simulink model "threeDOF"  (R2019b)
settings: Solver=ode3  StartTime=0.0  StopTime=inf  FixedStep=0.05  RelTol=1e-3  EnableMultiTasking=on
model workspace (MAT data in the model file):
  m = Simulink.Parameter
  m.Value = 2000
  m.DataType = 'auto'
  m.Dimensions = [1 1]
undefined symbols (not defined in the file): Angular, FrameId, FrameId_SL_Info, Linear, Seq, Stamp, X, Y, Z
libraries: robotlib x30, eeGeneralControl x1, vehdynlibsteering x1, autolibshared x1, sharedtransform x1
settings Model: ExplicitPartitioning=on  Creator=ivory  LastModifiedBy=ivory
settings DataIOCC: ReturnWorkspaceOutputs=off
settings OptimizationCC: StrengthReduction=on  PassReuseOutputArgsAs=Individual arguments  MaxStackSize=64  OptimizeBlockOrder=speed  OptimizationPriority=Speed  OptimizationCustomize=off  MultiThreadedLoops=on  EfficientTunableParamExpr=on
settings DebuggingCC: ParameterTunabilityLossMsg=error  ArithmeticOperatorsInVariantConditions=warning
settings HardwareCC: ProdBitPerPointer=32  ProdBitPerSizeT=32  ProdBitPerPtrDiffT=32  ProdLargestAtomicFloat=None  ProdIntDivRoundTo=Undefined  ProdEndianess=Unspecified  ProdWordSize=32  ProdHWDeviceType=Generic->Unspecified (assume 32-bit Generic)
settings SFSimCC: MATLABDynamicMemAlloc=off  CustomCodeUndefinedFunction=UseInterfaceOnly
settings RTWCC: SystemTargetFile=ert.tlc  HardwareBoard=Robot Operating System (ROS)  TLCOptions="-aInlineSetEventsForThisBaseRateFcn=TLC_FALSE -aSuppressMultiTaskScheduler=TLC_FALSE  -aRateBasedStepFcn=0"  TemplateMakefile=ert_default_tmf  GenerateReport=on  Toolchain=Catkin  IncludeHyperlinkInReport=on  LaunchReport=on  TargetLang=C++  GenerateTraceInfo=on  GenerateTraceReport=on  GenerateTraceReportSl=on  GenerateTraceReportSf=on  GenerateTraceReportEml=on
settings CodeAppCC: ForceParamTrailComments=on  IgnoreCustomStorageClasses=off  OperatorAnnotations=on  SimulinkDataObjDesc=on  SFDataObjDesc=on  InsertBlockDesc=on
settings ERTTargetCC: SupportContinuousTime=on  SupportVariableSizeSignals=on

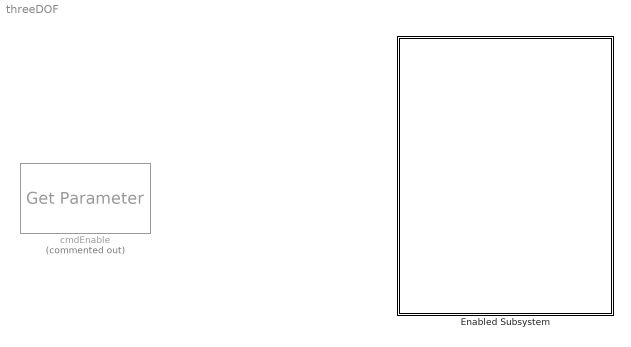
== system threeDOF ==
  Enabled Subsystem : Subsystem  TreatAsAtomicUnit=on
  cmdEnable : robotlib/Get Parameter  Commented=on  ParameterSource=Specify your own  ParameterName=/Enable  ParameterType=boolean  ParameterMaxArrayLength=16  ParameterInitialValue=false  SampleTime=-1  ShowErrorCodeOutput=off  ModelName=threeDOF  BlockId=ParamGet_threeDOF_291
      settings: SourceProductName=ROS Toolbox  SourceProductBaseCode=RR

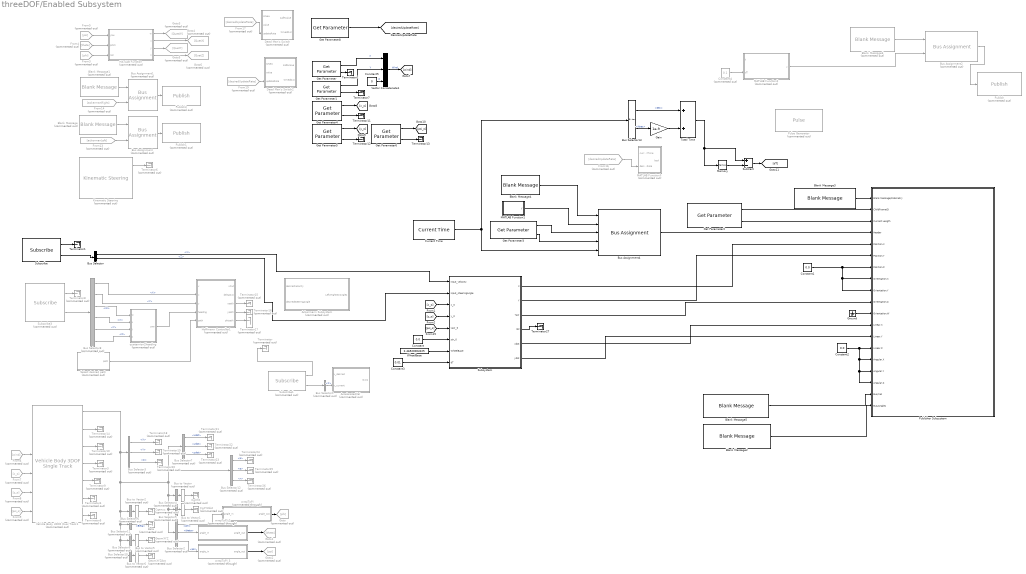
== system threeDOF/Enabled Subsystem ==
  AcceleratedVel : Subsystem  Commented=on
  Ackermann Subsystem : Subsystem  Commented=on
  Beta : Terminator  Commented=on
  Blank Message : robotlib/Blank Message  Commented=on  messageClass=Message  entityType=std_msgs/Float64  messageType=std_msgs/Float64  SampleTime=inf
      settings: SourceProductBaseCode=RO
  Blank Message1 : robotlib/Blank Message  Commented=on  messageClass=Message  entityType=std_msgs/Float64  messageType=std_msgs/Float64  SampleTime=inf
      settings: SourceProductBaseCode=RO
  Blank Message2 : robotlib/Blank Message  messageClass=Message  entityType=geometry_msgs/Point  messageType=geometry_msgs/Point  SampleTime=inf
      settings: SourceProductBaseCode=RO
  Blank Message3 : robotlib/Blank Message  messageClass=Message  entityType=nav_msgs/Odometry  messageType=nav_msgs/Odometry  SampleTime=inf
      settings: SourceProductBaseCode=RO
  Blank Message4 : robotlib/Blank Message  messageClass=Message  entityType=std_msgs/Header  messageType=std_msgs/Header  SampleTime=inf
      settings: SourceProductBaseCode=RO
  Blank Message5 : robotlib/Blank Message  messageClass=Message  entityType=geometry_msgs/Twist  messageType=geometry_msgs/Twist  SampleTime=inf
      settings: SourceProductBaseCode=RO
  Blank Message6 : robotlib/Blank Message  Commented=on  messageClass=Message  entityType=std_msgs/Float64  messageType=std_msgs/Float64  SampleTime=inf
      settings: SourceProductName=ROS Toolbox
  Bus Assignment : BusAssignment  Commented=on  AssignedSignals=Data
  Bus Assignment1 : BusAssignment  Commented=on  AssignedSignals=Data
  Bus Assignment2 : BusAssignment  Commented=on  AssignedSignals=Data
  Bus Assignment4 : BusAssignment  AssignedSignals=Seq,FrameId,FrameId_SL_Info.CurrentLength,Stamp
  Bus Selector : BusSelector  OutputSignals=Linear.X,Angular.Z
  Bus Selector1 : BusSelector  Commented=on  OutputSignals=Twist.Twist.Linear.X
  Bus Selector10 : BusSelector  Commented=on  OutputSignals=InertFrm.Geom.Vel.Xdot,InertFrm.Geom.Vel.Ydot,InertFrm.Geom.Vel.Zdot  OutputAsBus=on
  Bus Selector11 : BusSelector  Commented=on  OutputSignals=BdyFrm.Geom.Ang.Beta
  Bus Selector12 : BusSelector  Commented=on  OutputSignals=BdyFrm.Cg.AngVel.p,BdyFrm.Cg.AngVel.q,BdyFrm.Cg.AngVel.r
  Bus Selector13 : BusSelector  OutputSignals=Sec,Nsec
  Bus Selector2 : BusSelector  Commented=on  OutputSignals=InertFrm.Cg.Ang.phi,InertFrm.Cg.Ang.theta,InertFrm.Cg.Ang.psi
  Bus Selector3 : BusSelector  Commented=on  OutputSignals=InertFrm.Geom.Disp.X,InertFrm.Geom.Disp.Y,InertFrm.Geom.Disp.Z
  Bus Selector4 : BusSelector  Commented=on  OutputSignals=InertFrm.Cg.Disp.X,InertFrm.Cg.Disp.Y,InertFrm.Cg.Disp.Z  OutputAsBus=on
  Bus Selector5 : BusSelector  Commented=on  OutputSignals=InertFrm.Cg.Vel.Xdot,InertFrm.Cg.Vel.Ydot,InertFrm.Cg.Vel.Zdot  OutputAsBus=on
  Bus Selector6 : BusSelector  Commented=on  OutputSignals=BdyFrm.Cg.Acc.ax,BdyFrm.Cg.Acc.ay,BdyFrm.Cg.Acc.az  OutputAsBus=on
  Bus Selector7 : BusSelector  Commented=on  OutputSignals=BdyFrm.Cg.Vel.xdot,BdyFrm.Cg.Vel.ydot,BdyFrm.Cg.Vel.zdot
  Bus Selector8 : BusSelector  Commented=on  OutputSignals=Pose.Pose.Position.X,Pose.Pose.Position.Y,Pose.Pose.Orientation.W,Pose.Pose.Orientation.X,Pose.Pose.Orientation.Y,Pose.Pose.Orientation.Z
  Bus Selector9 : BusSelector  Commented=on  OutputSignals=InertFrm.Geom.Disp.X,InertFrm.Geom.Disp.Y,InertFrm.Geom.Disp.Z  OutputAsBus=on
  Bus to Vector{,1..2,5..6} (5 alike) : BusToVector  Commented=on
  CgXYZ : Terminator  Commented=on
  CgXYZdot : Terminator  Commented=on
  Cgaxyz : Terminator  Commented=on
  Constant : Constant  Value=0.0
  Constant1 : Constant  Value=0.0
  Constant2 : Constant  Value=0.0
  Constant3 : Constant  Value=0.01
  Constant4 : Constant  Commented=on  Value=0.1
  Constant5 : Constant  Value=0
  Current Time : robotlib/Current Time  OutputFormat=bus  SampleTime=-1  ModelName=threeDOF
      settings: SourceProductName=ROS Toolbox  SourceProductBaseCode=RR
  Dead Man's Switch : Subsystem  Commented=on  TreatAsAtomicUnit=on
  Dead Man's Switch2 : Subsystem  Commented=on  TreatAsAtomicUnit=on
  From13 : From  Commented=on  GotoTag=ackermanLeft
  From14 : From  Commented=on  GotoTag=ackermanRight
  From16 : From  Commented=on  GotoTag=desiredUpdateRate
  From17 : From  Commented=on  GotoTag=desiredUpdateRate
  From19 : From  Commented=on  GotoTag=desiredUpdateRate
  From3 : From  Commented=on  GotoTag=phi
  From4 : From  Commented=on  GotoTag=theta
  From5 : From  Commented=on  GotoTag=psi
  From6 : From  Commented=on  GotoTag=wind
  From7 : From  Commented=on  GotoTag=x_o
  From8 : From  Commented=on  GotoTag=y_o
  From9 : From  Commented=on  GotoTag=psi_o
  Gain : Gain  Gain=1e-9
  GeomXYZ : Terminator  Commented=on
  GeomXYZdot : Terminator  Commented=on
  Get Parameter : robotlib/Get Parameter  ParameterSource=Specify your own  ParameterName=windx  ParameterType=double  ParameterMaxArrayLength=16  ParameterInitialValue=0.0  SampleTime=-1  ShowErrorCodeOutput=on  ModelName=threeDOF  BlockId=ParamGet_threeDOF_199
      settings: SourceProductName=ROS Toolbox  SourceProductBaseCode=RR
  Get Parameter1 : robotlib/Get Parameter  ParameterSource=Specify your own  ParameterName=windy  ParameterType=double  ParameterMaxArrayLength=16  ParameterInitialValue=0.0  SampleTime=-1  ShowErrorCodeOutput=on  ModelName=threeDOF  BlockId=ParamGet_threeDOF_202
      settings: SourceProductName=ROS Toolbox  SourceProductBaseCode=RR
  Get Parameter2 : robotlib/Get Parameter  ParameterSource=Specify your own  ParameterName=childFrameId  ParameterType=uint8[] (string)  ParameterMaxArrayLength=128  ParameterInitialValue=uint8(['base_link'])  SampleTime=-1  ShowErrorCodeOutput=off  ModelName=threeDOF  BlockId=ParamGet_threeDOF_180
      settings: SourceProductName=ROS Toolbox  SourceProductBaseCode=RR
  Get Parameter3 : robotlib/Get Parameter  ParameterSource=Specify your own  ParameterName=headerFrameId  ParameterType=uint8[] (string)  ParameterMaxArrayLength=128  ParameterInitialValue=uint8(['odom'])  SampleTime=-1  ShowErrorCodeOutput=off  ModelName=threeDOF  BlockId=ParamGet_threeDOF_185
      settings: SourceProductName=ROS Toolbox  SourceProductBaseCode=RR
  Get Parameter4 : robotlib/Get Parameter  ParameterSource=Select from ROS network  ParameterName=x_init  ParameterType=double  ParameterMaxArrayLength=16  ParameterInitialValue=0.0  SampleTime=-1  ShowErrorCodeOutput=on  ModelName=threeDOF  BlockId=ParamGet_threeDOF_207
      settings: SourceProductName=ROS Toolbox  SourceProductBaseCode=RR
  Get Parameter5 : robotlib/Get Parameter  ParameterSource=Specify your own  ParameterName=y_init  ParameterType=double  ParameterMaxArrayLength=16  ParameterInitialValue=0.0  SampleTime=-1  ShowErrorCodeOutput=on  ModelName=threeDOF  BlockId=ParamGet_threeDOF_212
      settings: SourceProductName=ROS Toolbox  SourceProductBaseCode=RR
  Get Parameter6 : robotlib/Get Parameter  ParameterSource=Specify your own  ParameterName=psi_init  ParameterType=double  ParameterMaxArrayLength=16  ParameterInitialValue=0.0  SampleTime=-1  ShowErrorCodeOutput=on  ModelName=threeDOF  BlockId=ParamGet_threeDOF_215
      settings: SourceProductName=ROS Toolbox  SourceProductBaseCode=RR
  Get Parameter8 : robotlib/Get Parameter  ParameterSource=Specify your own  ParameterName=/desiredUpdateRate  ParameterType=double  ParameterMaxArrayLength=16  ParameterInitialValue=50  SampleTime=-1  ShowErrorCodeOutput=off  ModelName=threeDOF  BlockId=ParamGet_threeDOF_370
      settings: SourceProductName=ROS Toolbox  SourceProductBaseCode=RR
  Goto : Goto  Commented=on  GotoTag=phi
  Goto1 : Goto  Commented=on  GotoTag=theta
  Goto2 : Goto  Commented=on  GotoTag=psi
  Goto3 : Goto  Commented=on  GotoTag=QuetW
  Goto4 : Goto  Commented=on  GotoTag=QuetX
  Goto5 : Goto  Commented=on  GotoTag=QuetY
  Goto6 : Goto  Commented=on  GotoTag=QuetZ
  Ground : Ground
  Hoffmann Controller1 : Subsystem  Commented=on
  Kinematic Steering : vehdynlibsteering/Kinematic Steering  Commented=on  StrgType=Ackerman  StrgRatioType=Constant  Loc=Front  NrmlFctr=1  TrckWdth=1.0704  WhlBase=2.46520003225  Db=0  StrgRng=1.25*pi  StrgAngBpts="[-6.2832   -5.0265   -3.7699   -2.5133   -1.2566         0    1.2566    2.5133    3.7699    5.0265    6.2832]"  StrgRatioTbl=|  StrgRatio=18  StrgArmLngth=0.1  RckCsLngth=0.5  TieRodLngth=0.248  D=0.2  PnnRadius=0.0057  PnnRadiusTbl="[0.0055    0.0055    0.0056    0.0057    0.0058    0.0057    0.0057    0.0057    0.0056    0.0055    0.0055]"  RodLngth=0.1  ParaArmLngth=0.9  aMode=2
      | [13.5000   13.3750   13.2500   13.1250   13.0000   13.0000   13.0000   13.1250   13.2500   13.3750   13.5000
      | ]
      settings: SourceProductName=Vehicle Dynamics Blockset
  MATLAB Function : MATLAB Function  Commented=on  TreatAsAtomicUnit=on
  MATLAB Function1 : MATLAB Function  TreatAsAtomicUnit=on
  MATLAB Function2 : MATLAB Function  Commented=on  TreatAsAtomicUnit=on
  MATLAB Function3 : MATLAB Function  Commented=on  TreatAsAtomicUnit=on
  Memory : Memory
  Publish : robotlib/Publish  Commented=on  topicSource=Specify your own  topic=flag  messageType=std_msgs/Bool  messageQueueLength=1
      settings: SourceProductName=ROS Toolbox
  Publish1 : robotlib/Publish  Commented=on  topicSource=Specify your own  topic=ackermann_steer_left  messageType=std_msgs/Float64  messageQueueLength=1
      settings: SourceProductBaseCode=RO
  Publish3 : robotlib/Publish  Commented=on  topicSource=Specify your own  topic=ackermann_steer_right  messageType=std_msgs/Float64  messageQueueLength=1
      settings: SourceProductBaseCode=RO
  Publisher Subsystem : Subsystem
  Pulse Generator : DiscretePulseGenerator  Commented=on  PulseType=Time based  TimeSource=Use external signal  Period=1.0  PulseWidth=50%
  Select desired path : Subsystem  Commented=on
  Subscribe : robotlib/Subscribe  topicSource=Specify your own  topic=cmd_vel  messageType=geometry_msgs/Twist  sampleTime=-1  messageQueueLength=1
      settings: SourceProductBaseCode=RO
  Subscribe1 : robotlib/Subscribe  Commented=on  topicSource=Specify your own  topic=setvel  messageType=nav_msgs/Odometry  sampleTime=-1  messageQueueLength=1
      settings: SourceProductBaseCode=RO
  Subscribe3 : robotlib/Subscribe  Commented=on  topicSource=Specify your own  topic=odom  messageType=nav_msgs/Odometry  sampleTime=-1  messageQueueLength=1
      settings: SourceProductBaseCode=RO
  Subsystem : Subsystem
  Subtract : Sum  Inputs=+-
  Terminator{,3..6,8..10,14..26} (21 alike) : Terminator  Commented=on
  Terminator{1..2,7,11..13,27} (7 alike) : Terminator
  Total Time : Sum
  Vector Concatenate1 : Concatenate  NumInputs=3
  Vehicle Body 3DOF Dual Track1 : autolibshared/Vehicle Body 3DOF Single Track  Commented=on  trackMode=Dual  inputMode=External longitudinal velocity  frontSteerMode=on  rearSteerMode=off  windMode=on  muMode=off  extFMode=off  extMMode=off  extXo=on  extpsio=on  extxdoto=off  extro=off  extYo=on  extTamb=off  extydoto=off  aMode=2  NF=2  NR=2  m=2000  a=1.23260001612  b=1.23260001612  h=0.0  X_o=0  xdot_o=0  CalphaMode=off  sigmaMode=on  d=0  w=[1.0704,1.0704]  Cy_f=12e3  Cy_r=11e3  sigma_f=.1  sigma_r=.1  alpha_f_brk=[-.1 .1]  Cy_f_data=[-9e3 9e3]  alpha_r_brk=[-.1 .1]  Cy_r_data=[-9e3 9e3]  Y_o=0  ydot_o=0  Izz=4000  psi_o=0  r_o=0  Af=2  Cd=.3  Cl=.1  Cpm=.1  beta_w=[0:0.01:0.3]  Cs=[0:0.03:0.9]  Cym=[0:0.01:0.3]  Pabs=101325  Tair=273  g=9.81  mu=1  xdot_tol=.01  Fznom=5000  Fxtire_sat=7e4  Fytire_sat=7e4  longOff=0  latOff=0  vertOff=0  wrapAng=off
      settings: SourceProductName=Powertrain Blockset  SourceProductBaseCode=PW
  WheelBase : Constant  Value=2.46520003225
  quaternion2heading : Subsystem  Commented=on
  wrapToPI : MATLAB Function  Commented=through  TreatAsAtomicUnit=on
  wrapToPI_2 : MATLAB Function  Commented=through  TreatAsAtomicUnit=on
  wrapToPI_3 : MATLAB Function  Commented=through  TreatAsAtomicUnit=on
  wires:
  Get Parameter6/2 -> Terminator13/1
  From14/1 -> Bus Assignment1/2
  Blank Message/1 -> Bus Assignment/1
  Vector Concatenate1/1 -> [wind]  "Wind"
  Get Parameter1/2 -> Terminator7/1
  Get Parameter/1 -> Vector Concatenate1/1  "X"
  Bus Assignment1/1 -> Publish3/1
  Get Parameter/2 -> Terminator2/1
  From13/1 -> Bus Assignment/2
  Constant5/1 -> Vector Concatenate1/3  "Z"
  Get Parameter5/1 -> [y_o]
  Get Parameter1/1 -> Vector Concatenate1/2  "Y"
  Get Parameter5/2 -> Terminator12/1
  Get Parameter4/2 -> Terminator11/1
  Get Parameter4/1 -> [x_o]
  Get Parameter6/1 -> [psi_o]
  Blank Message1/1 -> Bus Assignment1/1
  Bus Assignment/1 -> Publish1/1
  Kinematic Steering/1 -> Terminator6/1
  MATLAB Function/1(w) -> Goto3/1
  MATLAB Function/3(y) -> Goto5/1
  MATLAB Function/2(x) -> Goto4/1
  From5/1 -> MATLAB Function/1(yaw)
  From3/1 -> MATLAB Function/3(roll)
  MATLAB Function/4(z) -> Goto6/1
  From4/1 -> MATLAB Function/2(pitch)
  Get Parameter8/1 -> [desiredUpdateRate]
  From17/1 -> Dead Man's Switch/3(updateRate)
  From19/1 -> Dead Man's Switch2/3(updateRate)
  Bus Selector3/3 -> Terminator20/1  "<Z>"
  Get Parameter3/2 -> Bus Assignment4/4
  Bus Selector8/1 -> Hoffmann Controller1/2(x)  "<X>"
  Hoffmann Controller1/3(xpath) -> Terminator15/1
  Blank Message5/1 -> Publisher Subsystem/18(Bus/Vel)
  Blank Message2/1 -> Publisher Subsystem/19(Bus/Angles)
  Subscribe1/2 -> Bus Selector1/1
  Bus Selector/1 -> Subsystem/1(input_velocity)  "<X>"
  Bus Selector6/1 -> Bus to Vector2/1
  Bus Selector8/2 -> Hoffmann Controller1/3(y)  "<Y>"
  Subscribe/2 -> Bus Selector/1
  Vehicle Body 3DOF Dual Track1/1 -> Bus Selector12/1, Bus Selector7/1, Bus Selector4/1, Bus Selector5/1, Bus Selector2/1, Bus Selector6/1, Bus Selector11/1, Bus Selector9/1, Bus Selector10/1, Bus Selector3/1
  Bus Selector7/1 -> Terminator21/1  "<xdot>"
  From9/1 -> Vehicle Body 3DOF Dual Track1/6
  Subscribe3/2 -> Bus Selector8/1
  wrapToPI/1(angle_out) -> Goto/1
  Constant1/1 -> Publisher Subsystem/9(Orientation.Y), Publisher Subsystem/8(Orientation.X), Publisher Subsystem/7(Position.Z)
  Bus Selector8/5 -> quaternion2heading/3(y)  "<Y>"
  Vehicle Body 3DOF Dual Track1/2 -> Terminator14/1
  Bus Assignment4/1 -> Publisher Subsystem/4(Header)
  Bus Selector7/2 -> Terminator22/1  "<ydot>"
  MATLAB Function2/1(y) -> Bus Assignment2/2
  Vehicle Body 3DOF Dual Track1/4 -> Terminator3/1
  Bus Selector7/3 -> Terminator23/1  "<zdot>"
  Bus Selector3/1 -> Terminator18/1  "<X>"
  Select desired path/1(path) -> Hoffmann Controller1/5(path)
  Bus Selector3/2 -> Terminator19/1  "<Y>"
  Bus Selector12/1 -> Terminator24/1  "<p>"
  Bus to Vector1/1 -> CgXYZdot/1
  Blank Message3/1 -> Publisher Subsystem/1(Blank Message/Odometry)
  From8/1 -> Vehicle Body 3DOF Dual Track1/5
  Ground/1 -> Publisher Subsystem/11(Orientation.W)
  Hoffmann Controller1/5(phipath) -> Terminator17/1
  From16/1 -> MATLAB Function3/2(desiredUpdateRate)
  Get Parameter2/2 -> Publisher Subsystem/3(Current Length)
  Bus Selector2/1 -> wrapToPI/1(angle_in)  "<phi>"
  Bus Selector2/3 -> wrapToPI_3/1(angle_in)  "<psi>"
  Bus to Vector/1 -> CgXYZ/1
  Gain/1 -> Total Time/2
  Total Time/1 -> Subtract/1, Memory/1
  From6/1 -> Vehicle Body 3DOF Dual Track1/3
  Bus to Vector6/1 -> GeomXYZdot/1
  Bus Selector11/1 -> Beta/1  "<Beta>"
  Bus Selector12/3 -> Terminator26/1  "<r>"
  Vehicle Body 3DOF Dual Track1/6 -> Terminator4/1
  Subscribe3/1 -> Terminator8/1
  Vehicle Body 3DOF Dual Track1/7 -> Terminator5/1
  Bus Selector10/1 -> Bus to Vector6/1
  quaternion2heading/1(yaw) -> Hoffmann Controller1/4(heading)
  Bus Selector12/2 -> Terminator25/1  "<q>"
  Bus to Vector2/1 -> Cgaxyz/1
  MATLAB Function1/1(y) -> Bus Assignment4/2
  wrapToPI_3/1(angle_out) -> Goto2/1
  Bus Selector13/1 -> Total Time/1  "<Sec>"
  From7/1 -> Vehicle Body 3DOF Dual Track1/4
  Subsystem/3(Yaw) -> Publisher Subsystem/10(Orientation.Z)
  Blank Message4/1 -> Bus Assignment4/1
  Vehicle Body 3DOF Dual Track1/5 -> Terminator9/1
  Bus Selector5/1 -> Bus to Vector1/1
  Bus Selector2/2 -> wrapToPI_2/1(angle_in)  "<theta>"
  Vehicle Body 3DOF Dual Track1/3 -> Terminator10/1
  Hoffmann Controller1/4(ypath) -> Terminator16/1
  Get Parameter3/1 -> Bus Assignment4/3
  Bus Selector9/1 -> Bus to Vector5/1
  Bus Selector8/3 -> quaternion2heading/1(w)  "<W>"
  Bus Selector1/1 -> AcceleratedVel/2(v_current)  "<X>"
  Bus Selector8/4 -> quaternion2heading/2(x)  "<X>"
  wrapToPI_2/1(angle_out) -> Goto1/1
  Current Time/1 -> Bus Assignment4/5, Bus Selector13/1
  Bus to Vector5/1 -> GeomXYZ/1
  Subscribe/1 -> Terminator1/1
  Bus Selector13/2 -> Gain/1  "<Nsec>"
  Get Parameter2/1 -> Publisher Subsystem/2(ChildFrameID)
  Bus Selector4/1 -> Bus to Vector/1
  Bus Selector8/6 -> quaternion2heading/4(z)  "<Z>"
  Subscribe1/1 -> Terminator/1
  Bus Selector/2 -> Subsystem/2(Input_steeringAngle)  "<Z>"
  [x_o] -> Subsystem/3(x_0)
  [y_o] -> Subsystem/4(y_0)
  [psi_o] -> Subsystem/5(yaw_0)
  WheelBase/1 -> Subsystem/7(WheelBase)
  Memory/1 -> Subtract/2
  Subtract/1 -> [dT]
  Constant/1 -> Subsystem/6(str_0)
  Subsystem/1(X) -> Publisher Subsystem/5(Position.X)
  Subsystem/2(Y) -> Publisher Subsystem/6(Position.Y)
  Subsystem/5(xdot) -> Publisher Subsystem/12(Linear.X)
  Subsystem/6(ydot) -> Publisher Subsystem/13(Linear.Y)
  Constant2/1 -> Publisher Subsystem/17(Angular.Z), Publisher Subsystem/16(Angular.Y), Publisher Subsystem/15(Angular.X), Publisher Subsystem/14(Linear.Z)
  Subsystem/4(Str) -> Terminator27/1
  Constant3/1 -> Subsystem/8(dT)
  Blank Message6/1 -> Bus Assignment2/1
  Bus Assignment2/1 -> Publish/1
  Constant4/1 -> MATLAB Function2/2(dT)

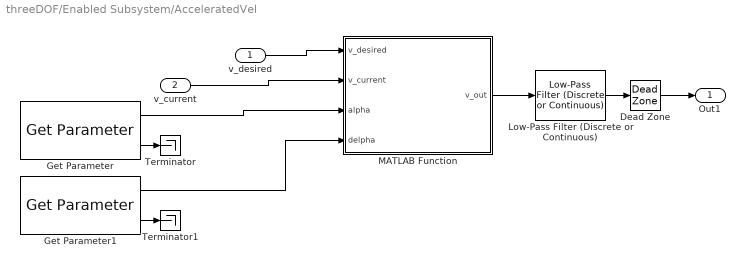
== system threeDOF/Enabled Subsystem/AcceleratedVel ==
  v_desired : Inport
  v_current : Inport  Port=2
  Dead Zone : DeadZone  LowerValue=-0.05  UpperValue=0.05  SaturateOnIntegerOverflow=on
  Get Parameter : robotlib/Get Parameter  ParameterSource=Specify your own  ParameterName=alpha  ParameterType=double  ParameterMaxArrayLength=16  ParameterInitialValue=1.5  SampleTime=-1  ShowErrorCodeOutput=on  ModelName=threeDOF  BlockId=ParamGet_threeDOF_94
      settings: SourceProductName=Robotics System Toolbox  SourceProductBaseCode=RO
  Get Parameter1 : robotlib/Get Parameter  ParameterSource=Specify your own  ParameterName=delpha  ParameterType=double  ParameterMaxArrayLength=16  ParameterInitialValue=-1.5  SampleTime=-1  ShowErrorCodeOutput=on  ModelName=threeDOF  BlockId=ParamGet_threeDOF_96
      settings: SourceProductName=Robotics System Toolbox  SourceProductBaseCode=RO
  Low-Pass Filter (Discrete or Continuous) : eeGeneralControl/Low-Pass Filter (Discrete or Continuous)  K=1  T=0.89  B=inf  A=-inf  Ts=-1
      settings: SourceProductName=Simscape Electrical
  MATLAB Function : MATLAB Function  TreatAsAtomicUnit=on
  Terminator : Terminator
  Terminator1 : Terminator
  Out1 : Outport  VectorParamsAs1DForOutWhenUnconnected=off
  wires:
  v_desired/1 -> MATLAB Function/1(v_desired)
  v_current/1 -> MATLAB Function/2(v_current)
  Get Parameter/1 -> MATLAB Function/3(alpha)
  Get Parameter/2 -> Terminator/1
  Get Parameter1/2 -> Terminator1/1
  Get Parameter1/1 -> MATLAB Function/4(delpha)
  Dead Zone/1 -> Out1/1
  MATLAB Function/1(v_out) -> Low-Pass Filter (Discrete or Continuous)/1
  Low-Pass Filter (Discrete or Continuous)/1 -> Dead Zone/1

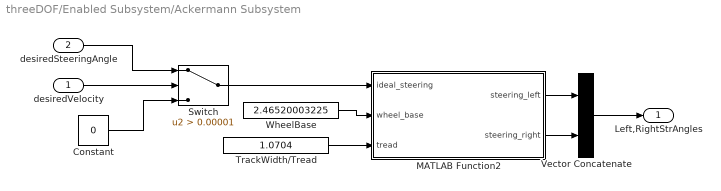
== system threeDOF/Enabled Subsystem/Ackermann Subsystem ==
  desiredVelocity : Inport
  desiredSteeringAngle : Inport  Port=2
  Constant : Constant  Value=0
  MATLAB Function2 : MATLAB Function  TreatAsAtomicUnit=on
  Switch : Switch  Criteria=u2 > Threshold  Threshold=0.00001
  TrackWidth/Tread : Constant  Value=1.0704
  Vector Concatenate : Concatenate
  WheelBase : Constant  Value=2.46520003225
  Left,RightStrAngles : Outport  VectorParamsAs1DForOutWhenUnconnected=off
  wires:
  Switch/1 -> MATLAB Function2/1(ideal_steering)
  TrackWidth/Tread/1 -> MATLAB Function2/3(tread)
  Constant/1 -> Switch/3
  desiredVelocity/1 -> Switch/2
  WheelBase/1 -> MATLAB Function2/2(wheel_base)
  MATLAB Function2/1(steering_left) -> Vector Concatenate/1
  MATLAB Function2/2(steering_right) -> Vector Concatenate/2
  desiredSteeringAngle/1 -> Switch/1
  Vector Concatenate/1 -> Left,RightStrAngles/1

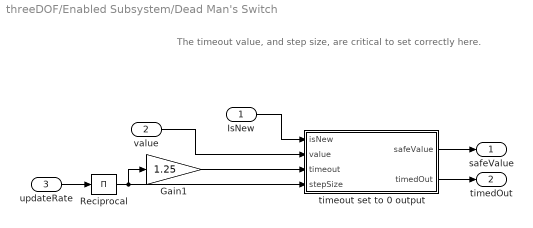
== system threeDOF/Enabled Subsystem/Dead Man's Switch ==
  note: The timeout value, and step size, are critical to set correctly here.
  IsNew : Inport
  value : Inport  Port=2
  updateRate : Inport  Port=3
  Gain1 : Gain  Gain=1.25
  Reciprocal : Product  Inputs=1
  timeout set to 0 output : MATLAB Function  TreatAsAtomicUnit=on
  safeValue : Outport  InitialOutput=[0]  VectorParamsAs1DForOutWhenUnconnected=off
  timedOut : Outport  Port=2  InitialOutput=[0]  VectorParamsAs1DForOutWhenUnconnected=off
  wires:
  IsNew/1 -> timeout set to 0 output/1(isNew)
  timeout set to 0 output/1(safeValue) -> safeValue/1
  value/1 -> timeout set to 0 output/2(value)
  Gain1/1 -> timeout set to 0 output/3(timeout)
  timeout set to 0 output/2(timedOut) -> timedOut/1
  Reciprocal/1 -> Gain1/1, timeout set to 0 output/4(stepSize)
  updateRate/1 -> Reciprocal/1

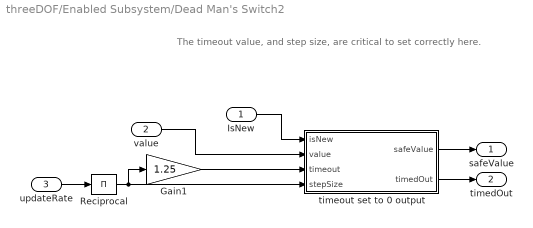
== system threeDOF/Enabled Subsystem/Dead Man's Switch2 ==
  note: The timeout value, and step size, are critical to set correctly here.
  IsNew : Inport
  value : Inport  Port=2
  updateRate : Inport  Port=3
  Gain1 : Gain  Gain=1.25
  Reciprocal : Product  Inputs=1
  timeout set to 0 output : MATLAB Function  TreatAsAtomicUnit=on
  safeValue : Outport  InitialOutput=[0]  VectorParamsAs1DForOutWhenUnconnected=off
  timedOut : Outport  Port=2  InitialOutput=[0]  VectorParamsAs1DForOutWhenUnconnected=off
  wires:
  IsNew/1 -> timeout set to 0 output/1(isNew)
  timeout set to 0 output/1(safeValue) -> safeValue/1
  value/1 -> timeout set to 0 output/2(value)
  Gain1/1 -> timeout set to 0 output/3(timeout)
  timeout set to 0 output/2(timedOut) -> timedOut/1
  Reciprocal/1 -> Gain1/1, timeout set to 0 output/4(stepSize)
  updateRate/1 -> Reciprocal/1

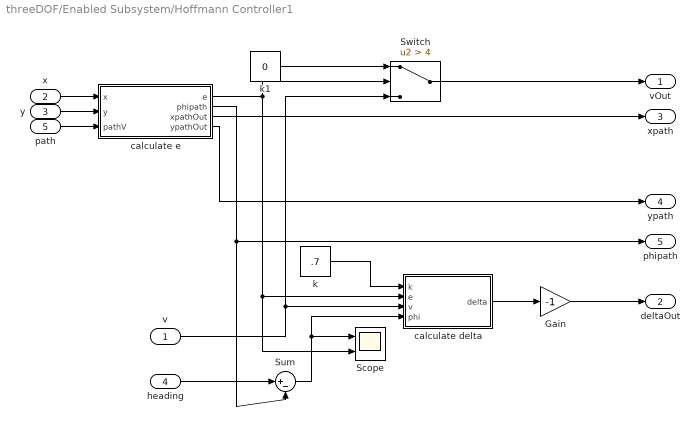
== system threeDOF/Enabled Subsystem/Hoffmann Controller1 ==
  v : Inport
  x : Inport  Port=2
  y : Inport  Port=3
  heading : Inport  Port=4
  path : Inport  Port=5
  Gain : Gain  Gain=-1
  Scope : Scope  NumInputPorts=2
  Sum : Sum  Inputs=|+-
  Switch : Switch  Criteria=u2 > Threshold  Threshold=4
  calculate delta : MATLAB Function  TreatAsAtomicUnit=on
  calculate e : MATLAB Function  TreatAsAtomicUnit=on
  k : Constant  Value=.7
  k1 : Constant  Value=0
  vOut : Outport  VectorParamsAs1DForOutWhenUnconnected=off
  deltaOut : Outport  Port=2  VectorParamsAs1DForOutWhenUnconnected=off
  xpath : Outport  Port=3  VectorParamsAs1DForOutWhenUnconnected=off
  ypath : Outport  Port=4  VectorParamsAs1DForOutWhenUnconnected=off
  phipath : Outport  Port=5  VectorParamsAs1DForOutWhenUnconnected=off
  wires:
  v/1 -> Switch/3, calculate delta/3(v)
  path/1 -> calculate e/3(pathV)
  x/1 -> calculate e/1(x)
  y/1 -> calculate e/2(y)
  calculate e/2(phipath) -> phipath/1, Sum/2
  calculate e/1(e) -> Switch/2, Scope/2, calculate delta/2(e)
  Sum/1 -> Scope/1, calculate delta/4(phi)
  k/1 -> calculate delta/1(k)
  calculate e/3(xpathOut) -> xpath/1
  calculate e/4(ypathOut) -> ypath/1
  Switch/1 -> vOut/1
  k1/1 -> Switch/1
  heading/1 -> Sum/1
  calculate delta/1(delta) -> Gain/1
  Gain/1 -> deltaOut/1

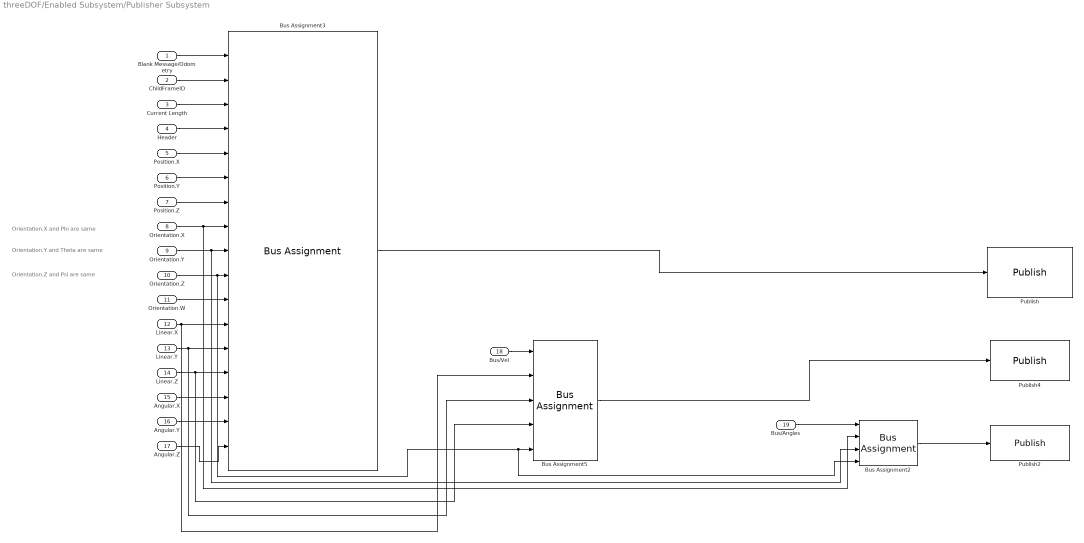
== system threeDOF/Enabled Subsystem/Publisher Subsystem ==
  note: Orientation.X and Phi are same
  note: Orientation.Y and Theta are same
  note: Orientation.Z and Psi are same
  Blank Message/Odometry : Inport
  ChildFrameID : Inport  Port=2
  Current Length : Inport  Port=3
  Header : Inport  Port=4
  Position.X : Inport  Port=5
  Position.Y : Inport  Port=6
  Position.Z : Inport  Port=7
  Orientation.X : Inport  Port=8
  Orientation.Y : Inport  Port=9
  Orientation.Z : Inport  Port=10
  Orientation.W : Inport  Port=11
  Linear.X : Inport  Port=12
  Linear.Y : Inport  Port=13
  Linear.Z : Inport  Port=14
  Angular.X : Inport  Port=15
  Angular.Y : Inport  Port=16
  Angular.Z : Inport  Port=17
  Bus/Vel : Inport  Port=18
  Bus/Angles : Inport  Port=19
  Bus Assignment2 : BusAssignment  AssignedSignals=X,Y,Z
  Bus Assignment3 : BusAssignment  AssignedSignals=ChildFrameId,ChildFrameId_SL_Info.CurrentLength,Header,Pose.Pose.Position.X,Pose.Pose.Position.Y,Pose.Pose.Position.Z,Pose.Pose.Orientation.X,Pose.Pose.Orientation.Y,Pose.Pose.Orientation.Z,Pose.Pose.Orientation.W,Twist.Twist.Linear.X,Twist.Twist.Linear.Y,Twist.Twist.Linear.Z,Twist.Twist.Angular.X,Twist.Twist.Angular.Y,Twist.Twist.Angular.Z
  Bus Assignment5 : BusAssignment  AssignedSignals=Linear.X,Linear.Y,Linear.Z,Angular.Z
  Publish : robotlib/Publish  topicSource=Specify your own  topic=setvel  messageType=nav_msgs/Odometry  messageQueueLength=1
      settings: SourceProductBaseCode=RO
  Publish2 : robotlib/Publish  topicSource=Specify your own  topic=angles  messageType=geometry_msgs/Point  messageQueueLength=1
      settings: SourceProductBaseCode=RO
  Publish4 : robotlib/Publish  topicSource=Specify your own  topic=vel  messageType=geometry_msgs/Twist  messageQueueLength=1
      settings: SourceProductBaseCode=RO
  wires:
  Bus Assignment2/1 -> Publish2/1
  Bus Assignment3/1 -> Publish/1
  Bus Assignment5/1 -> Publish4/1
  Blank Message/Odometry/1 -> Bus Assignment3/1
  ChildFrameID/1 -> Bus Assignment3/2
  Current Length/1 -> Bus Assignment3/3
  Header/1 -> Bus Assignment3/4
  Position.X/1 -> Bus Assignment3/5
  Position.Y/1 -> Bus Assignment3/6
  Position.Z/1 -> Bus Assignment3/7
  Orientation.W/1 -> Bus Assignment3/11
  Linear.X/1 -> Bus Assignment5/2, Bus Assignment3/12
  Linear.Y/1 -> Bus Assignment5/3, Bus Assignment3/13
  Linear.Z/1 -> Bus Assignment5/4, Bus Assignment3/14
  Angular.X/1 -> Bus Assignment3/15
  Angular.Y/1 -> Bus Assignment3/16
  Angular.Z/1 -> Bus Assignment3/17
  Bus/Vel/1 -> Bus Assignment5/1
  Orientation.Z/1 -> Bus Assignment2/4, Bus Assignment5/5, Bus Assignment3/10
  Orientation.X/1 -> Bus Assignment2/2, Bus Assignment3/8
  Orientation.Y/1 -> Bus Assignment2/3, Bus Assignment3/9
  Bus/Angles/1 -> Bus Assignment2/1

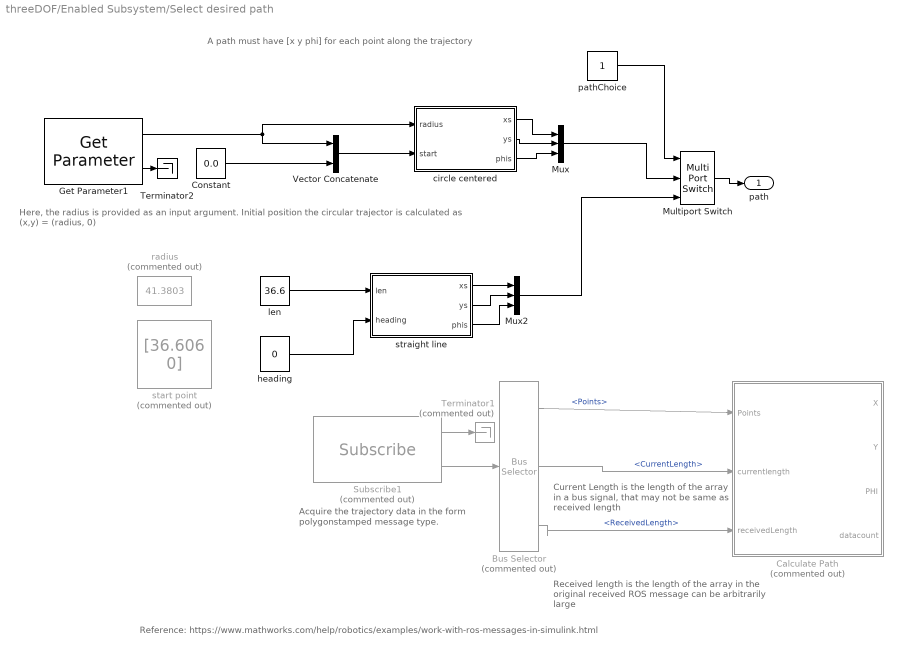
== system threeDOF/Enabled Subsystem/Select desired path ==
  note: Here, the radius is provided as an input argument. Initial position the circular trajector is calculated as (x,y) = (radius, 0)
  note: Reference: https://www.mathworks.com/help/robotics/examples/work-with-ros-messages-in-simulink.html
  note: Received length is the length of the array in
      | the original received ROS message can
      | be arbitrarily large
  note: Current Length is the length of the array in a bus signal, that may not be same as received length
  note: Acquire the trajectory data in the form polygonstamped message type.
  note: A path must have [x y phi] for each point along the trajectory
  Bus Selector : BusSelector  Commented=on  OutputSignals=Polygon.Points,Polygon.Points_SL_Info.CurrentLength,Polygon.Points_SL_Info.ReceivedLength
  Calculate Path : MATLAB Function  Commented=on  TreatAsAtomicUnit=on
  Constant : Constant  Value=0.0
  Get Parameter1 : robotlib/Get Parameter  ParameterSource=Specify your own  ParameterName=radius  ParameterType=double  ParameterMaxArrayLength=16  ParameterInitialValue=41.3803  SampleTime=-1  ShowErrorCodeOutput=on  ModelName=threeDOF  BlockId=ParamGet_threeDOF_326
      settings: SourceProductName=Robotics System Toolbox  SourceProductBaseCode=RO
  Multiport Switch : MultiPortSwitch  Inputs=2
  Mux : Mux  Inputs=3
  Mux2 : Mux  Inputs=3
  Subscribe1 : robotlib/Subscribe  Commented=on  topicSource=Select from ROS network  topic=/trajectory  messageType=geometry_msgs/PolygonStamped  sampleTime=-1  messageQueueLength=1
      settings: SourceProductBaseCode=RO
  Terminator1 : Terminator  Commented=on
  Terminator2 : Terminator
  Vector Concatenate : Concatenate
  circle centered : MATLAB Function  TreatAsAtomicUnit=on
  heading : Constant  Value=0
  len : Constant  Value=36.6
  "pathChoice " : Constant
  radius : Constant  Commented=on  Value=41.3803
  start point : Constant  Commented=on  Value=[36.606 0]
  straight line : MATLAB Function  TreatAsAtomicUnit=on
  path : Outport  VectorParamsAs1DForOutWhenUnconnected=off
  wires:
  Subscribe1/1 -> Terminator1/1
  Subscribe1/2 -> Bus Selector/1
  Bus Selector/1 -> Calculate Path/1(Points)  "<Points>"
  Bus Selector/2 -> Calculate Path/2(currentlength)  "<CurrentLength>"
  Bus Selector/3 -> Calculate Path/3(receivedLength)  "<ReceivedLength>"
  straight line/2(ys) -> Mux2/2
  "pathChoice "/1 -> Multiport Switch/1
  Multiport Switch/1 -> path/1
  straight line/1(xs) -> Mux2/1
  circle centered/3(phis) -> Mux/3
  len/1 -> straight line/1(len)
  heading/1 -> straight line/2(heading)
  circle centered/1(xs) -> Mux/1
  circle centered/2(ys) -> Mux/2
  Mux2/1 -> Multiport Switch/3
  Mux/1 -> Multiport Switch/2
  straight line/3(phis) -> Mux2/3
  Vector Concatenate/1 -> circle centered/2(start)
  Get Parameter1/2 -> Terminator2/1
  Get Parameter1/1 -> circle centered/1(radius), Vector Concatenate/1
  Constant/1 -> Vector Concatenate/2

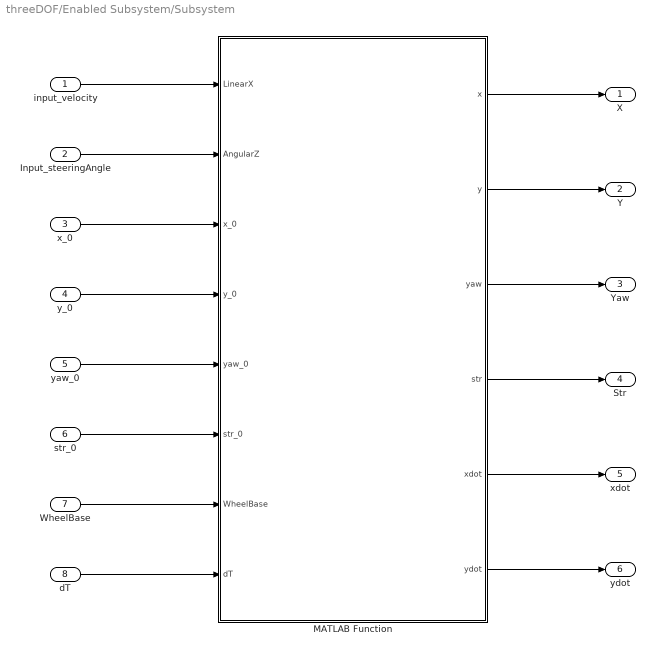
== system threeDOF/Enabled Subsystem/Subsystem ==
  input_velocity : Inport
  Input_steeringAngle : Inport  Port=2
  x_0 : Inport  Port=3
  y_0 : Inport  Port=4
  yaw_0 : Inport  Port=5
  str_0 : Inport  Port=6
  WheelBase : Inport  Port=7
  dT : Inport  Port=8
  MATLAB Function : MATLAB Function  TreatAsAtomicUnit=on
  X : Outport  VectorParamsAs1DForOutWhenUnconnected=off
  Y : Outport  Port=2  VectorParamsAs1DForOutWhenUnconnected=off
  Yaw : Outport  Port=3  VectorParamsAs1DForOutWhenUnconnected=off
  Str : Outport  Port=4  VectorParamsAs1DForOutWhenUnconnected=off
  xdot : Outport  Port=5  VectorParamsAs1DForOutWhenUnconnected=off
  ydot : Outport  Port=6  VectorParamsAs1DForOutWhenUnconnected=off
  wires:
  input_velocity/1 -> MATLAB Function/1(LinearX)
  Input_steeringAngle/1 -> MATLAB Function/2(AngularZ)
  x_0/1 -> MATLAB Function/3(x_0)
  y_0/1 -> MATLAB Function/4(y_0)
  yaw_0/1 -> MATLAB Function/5(yaw_0)
  str_0/1 -> MATLAB Function/6(str_0)
  WheelBase/1 -> MATLAB Function/7(WheelBase)
  MATLAB Function/1(x) -> X/1
  MATLAB Function/2(y) -> Y/1
  MATLAB Function/3(yaw) -> Yaw/1
  MATLAB Function/4(str) -> Str/1
  MATLAB Function/5(xdot) -> xdot/1
  MATLAB Function/6(ydot) -> ydot/1
  dT/1 -> MATLAB Function/8(dT)

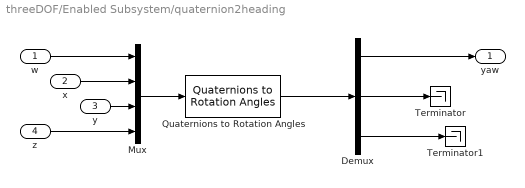
== system threeDOF/Enabled Subsystem/quaternion2heading ==
  w : Inport
  x : Inport  Port=2
  y : Inport  Port=3
  z : Inport  Port=4
  Demux : Demux  Outputs=3
  Mux : Mux
  Quaternions to Rotation Angles : sharedtransform/Quaternions to Rotation Angles  rotationOrder=ZYX  aMode=aMode
      settings: SourceProductBaseCode=AE
  Terminator : Terminator
  Terminator1 : Terminator
  yaw : Outport  VectorParamsAs1DForOutWhenUnconnected=off
  wires:
  Quaternions to Rotation Angles/1 -> Demux/1
  Demux/2 -> Terminator/1
  Demux/3 -> Terminator1/1
  Demux/1 -> yaw/1
  w/1 -> Mux/1
  x/1 -> Mux/2
  y/1 -> Mux/3
  z/1 -> Mux/4
  Mux/1 -> Quaternions to Rotation Angles/1

== matlab function threeDOF/Enabled Subsystem/MATLAB Function ==
  data: w output; x output; yaw input; y output; pitch input; roll input; z output
function [w, x, y, z] = rpyToQueternion(yaw, pitch, roll)


    cy = cos(yaw * 0.5);
    sy = sin(yaw * 0.5);
    cp = cos(pitch * 0.5);
    sp = sin(pitch * 0.5);
    cr = cos(roll * 0.5);
    sr = sin(roll * 0.5);


    w = cy * cp * cr + sy * sp * sr;
    x = cy * cp * sr - sy * sp * cr;
    y = sy * cp * sr + cy * sp * cr;
    z = sy * cp * cr - cy * sp * sr;

end

== matlab function threeDOF/Enabled Subsystem/AcceleratedVel/MATLAB Function ==
  settings: updateMethod=DISCRETE
  data: v_desired input; v_out output; v_current input; alpha input; delpha input
function v_out = AcceleratedVel(v_desired, v_current, alpha, delpha)

persistent init_flag
if isempty(init_flag)
    init_flag = 0;
    v_out = 0;
    return;
end

if(init_flag == 0)
    v_current = 0; %Car has not yet started.
end

dt = 0.01;
v_epsilon = 0.05;

if(v_current < v_desired+v_epsilon) %if current velocity is less than desired velocity, accelerate
    v_out = max(v_desired, v_current + alpha*dt);
elseif(v_current > v_desired + v_epsilon)
    v_out = min(v_desired, v_current + delpha*dt);
else
    v_out = v_desired;
end

== matlab function threeDOF/Enabled Subsystem/MATLAB Function1 ==
  data: y output
function y = counter

persistent count;

if isempty(count)
  count = uint32(0);
end

count  = count+1;

y = count;

== matlab function threeDOF/Enabled Subsystem/wrapToPI ==
  data: angle_in input; angle_out output
function angle_out = wrapToPIWrapper(angle_in)

% We need to constrain angles within [-pi, pi]

% angle_out = wrapToPi(angle_in);


angle_out = rem (angle_in, 2*pi);
idx = find (abs (angle_out) > pi);
angle_out(idx) = angle_out(idx) - 2*pi * sign (angle_out(idx));

== matlab function threeDOF/Enabled Subsystem/wrapToPI_2 ==
  data: angle_in input; angle_out output
function angle_out = wrapToPIWrapper(angle_in)

% We need to constrain angles within [-pi, pi]

% angle_out = wrapToPi(angle_in);


angle_out = rem (angle_in, 2*pi);
idx = find (abs (angle_out) > pi);
angle_out(idx) = angle_out(idx) - 2*pi * sign (angle_out(idx));

== matlab function threeDOF/Enabled Subsystem/wrapToPI_3 ==
  data: angle_in input; angle_out output
function angle_out = wrapToPIWrapper(angle_in)

% We need to constrain angles within [-pi, pi]

% angle_out = wrapToPi(angle_in);


angle_out = rem (angle_in, 2*pi);
idx = find (abs (angle_out) > pi);
angle_out(idx) = angle_out(idx) - 2*pi * sign (angle_out(idx));

== matlab function threeDOF/Enabled Subsystem/Ackermann Subsystem/MATLAB Function2 ==
  data: ideal_steering input; steering_left output; wheel_base input; tread input; steering_right output
function [steering_left, steering_right] = Ackermann(ideal_steering, wheel_base, tread)

turning_radius = wheel_base/tan(ideal_steering);

steering_left = atan(wheel_base/( turning_radius - tread/2) );

steering_right = atan(wheel_base/( turning_radius + tread/2) );

== matlab function threeDOF/Enabled Subsystem/Select desired path/Calculate Path ==
  data: X output size=32000; Points input Bus: SL_Bus_hoffmansubsystem_geometry_msgs_Point32 size=8000 [0..32000]; currentlength input; Y output size=32000; PHI output size=32000; datacount output; receivedLength input
function [X, Y,PHI,datacount] = fcn(Points, currentlength, receivedLength)
%#codegen


X = zeros(8000,1);
Y = zeros(8000,1);
PHI = zeros(8000,1);

%We will work on array using the current Length as, Simulink might
%truncate an arbitrarily large according to the maximum length set


for i = 1:currentlength
        %Points(i).X
        %Points(i).Y
        X(i) = Points(i).X;
        Y(i) = Points(i).Y;

        %We will calculate current headway as the instantaneous slope
        if ( i > 1)
           % atan2((Y(i) - Y(i-1)),(X(i) - X(i-1)))
           PHI(i) = atan2((Y(i) - Y(i-1)),(X(i) - X(i-1)));
        else
           PHI(i) = 0;
        end
end
X(i+1) =  Points(1).X;
Y(i+1) = Points(1).Y;
PHI(i+1) = atan2((Y(1) - Y(i)),(X(1) - X(i)));

datacount = double(currentlength+1);
end

== matlab function threeDOF/Enabled Subsystem/Hoffmann Controller1/calculate delta ==
  data: delta output; k input; e input; v input; phi input
function delta = fcn(k,e,v,phi)
%#codegen
if( abs(v) < eps )
    v = eps;
end

% if phi is greater than pi (or less than -pi), then 
% we normalize to between [-pi,pi]
if( phi < -pi )
    phi = phi+2*pi;
elseif( phi > pi )
    phi = phi-2*pi;
end

delta = phi + atan2(k*e,v);

== matlab function threeDOF/Enabled Subsystem/Hoffmann Controller1/calculate e ==
  data: e output; x input; y input; pathV input; phipath output; xpathOut output; ypathOut output
function [e,phipath,xpathOut,ypathOut] = fcn(x,y,pathV)
%#codegen
path=reshape(pathV,[],3);
x1 = path(1,1);
y1 = path(1,2);
phi1=path(1,3);
etmp = inf;
e = inf;
index=1;
% find the nearest x,y
for i=1:length(path)
   etmp = sqrt((x-path(i,1))^2+(y-path(i,2))^2);
   if( etmp < e )
       e = etmp;
       index=i;
   end
end

xpathOut=path(index,1);
ypathOut=path(index,2);
phipath=path(index,3);

ex1 = (path(index,1)-x);
ey1 = (path(index,2)-y);
ex2 = cos(phipath);
ey2 = sin(phipath);
sinnnn = ex1*ey2-ey1*ex2;
e = sign(sinnnn)*e;

== matlab function threeDOF/Enabled Subsystem/Select desired path/circle centered ==
  data: xs output; radius input; start input; ys output; phis output
function [xs,ys,phis] = fcn(radius,start)
%#codegen
angles=linspace(-pi,pi,3001);
r = radius*exp(angles*1j);
xs = real(r)-radius+start(1);
ys = imag(r)+start(2);
phis=(pi/2)+angles;

% % To visualize the angles, run this code:
% radius=3.6; start=[0 0];
% angles=linspace(-pi,pi,300);
% r = radius*exp(angles*1j);
% xs = real(r)-radius+start(1);
% ys = imag(r)+start(2);
% % since the direction of travel is in the 'x' direction, the 
% % heading (phi) matchines the angle of the circle
% phis=(pi/2)+angles;
% xends=cos(phis);yends=sin(phis);
% figure;plot(xs,ys);hold on; quiver(xs,ys,xends,yends);axis equal;hold off

== matlab function threeDOF/Enabled Subsystem/Select desired path/straight line ==
  data: xs output; len input; heading input; ys output; phis output
function [xs,ys,phis] = fcn(len,heading)
%#codegen
r = linspace(0,len,3001);
xs = r*cos(heading);
ys = r*sin(heading);
phis = heading*ones(1,length(r));

== matlab function threeDOF/Enabled Subsystem/MATLAB Function3 ==
  settings: updateMethod=DISCRETE
  data: currentTime input; bool output; desiredUpdateRate input
function bool = enable(currentTime, desiredUpdateRate)

    persistent oldTime
    if isempty(oldTime)
        oldTime = currentTime;
    end

    if( currentTime - oldTime < (1/desiredUpdateRate)  )
        bool = false;
    else
        bool = true;
        oldTime = currentTime;
    end

== matlab function threeDOF/Enabled Subsystem/Dead Man's Switch/timeout set to 0 output ==
  settings: updateMethod=DISCRETE
  data: isNew input; safeValue output; value input; timeout input; timedOut output; stepSize input
function [safeValue,timedOut] = fcn(isNew,value,timeout,stepSize)
%#codegen
persistent sinceLastMsg
timedOut=true;
if isempty(sinceLastMsg)
    sinceLastMsg=(timeout/stepSize)+1;
end

safeValue=0;
% if no new message
% after timeout, we output 0
if( isNew == true )
    sinceLastMsg = 0;
else
    sinceLastMsg = sinceLastMsg+1;
end

% Note: we require step size as an input here, and depend on our
% system being executed at a regular rate, or bad things will happen
if( sinceLastMsg < timeout/stepSize )
    timedOut = false;
end
    
if( timedOut == false )
    safeValue = value;
end

== matlab function threeDOF/Enabled Subsystem/Subsystem/MATLAB Function ==
  data: x output; y output; LinearX input; AngularZ input; x_0 input; y_0 input; yaw_0 input; yaw output; str_0 input; WheelBase input; str output; xdot output; ydot output; dT input
function [x, y, yaw, str, xdot, ydot] = BicycleModel(LinearX,  AngularZ, x_0, y_0, yaw_0, str_0, WheelBase, dT)

    persistent x_old y_old yaw_old str_old

    if isempty(x_old)
        x_old = x_0;
    end
    
    if isempty(y_old)
        y_old = y_0;
    end
    
    if isempty(yaw_old)
        yaw_old = yaw_0;
    end
    
    if isempty(str_old)
        str_old = str_0;
    end
    
    % Rate of change of tire angle
    u2 = (AngularZ - str_old)/dT;
    
    xdot = LinearX*cos(str_old)*cos(yaw_old);
    ydot = LinearX*cos(str_old)*sin(yaw_old);
    x = x_old + dT*xdot;
    y = y_old + dT*ydot;
    
    str = str_old + dT*u2;
    
    if(str >0.5236)
        str = 0.5236;
    end
    
    if(str < - 0.5236)
        str = -0.5236;
    end
    
    yaw = yaw_old + dT*LinearX*(1/WheelBase)*sin(str_old);
    
    while(yaw < 0)
        yaw = yaw + 2*pi;
    end
    
    while(yaw > 2*pi)
        yaw = yaw - 2*pi;
    end
    
    x_old = x;
    y_old = y;
    str_old = str;
    yaw_old = yaw;
  
end

== matlab function threeDOF/Enabled Subsystem/MATLAB Function2 ==
  data: t input; y output; dT input
function y = fcn(t, dT)

persistent onoff
if isempty(onoff)
    onoff = 0.0;
end

persistent oldtime

persistent timediff

if isempty(timediff)
    timediff = 0.0;
end

if isempty(oldtime)
    oldtime = t;
    onoff = 0.0;
    
else
    if timediff >= dT
        onoff = 1.0;
        oldtime = t;
    else
        timediff = t - oldtime;
        onoff = 0.0;
    end
end

y = onoff;        
end

== matlab function threeDOF/Enabled Subsystem/Dead Man's Switch2/timeout set to 0 output ==
  settings: updateMethod=DISCRETE
  data: isNew input; safeValue output; value input; timeout input; timedOut output; stepSize input
function [safeValue,timedOut] = fcn(isNew,value,timeout,stepSize)
%#codegen
persistent sinceLastMsg
timedOut=true;
if isempty(sinceLastMsg)
    sinceLastMsg=(timeout/stepSize)+1;
end

safeValue=0;
% if no new message
% after timeout, we output 0
if( isNew == true )
    sinceLastMsg = 0;
else
    sinceLastMsg = sinceLastMsg+1;
end

% Note: we require step size as an input here, and depend on our
% system being executed at a regular rate, or bad things will happen
if( sinceLastMsg < timeout/stepSize )
    timedOut = false;
end
    
if( timedOut == false )
    safeValue = value;
end
